simulink model "basic_cosimulation_c_1_sm_master"  (R2021b)
settings: Solver=ode4  StartTime=0.0  StopTime=inf  FixedStep=5e-05  RelTol=1e-3  EnableMultiTasking=on
PostLoadFcn:
  | %
  | % Script for validation of swtiching model design with it's respective
  | % average model.
  | %
  | % Here it is presented the design of the inverter to the 6 kW Fuel Cell
  | % model.
  | 
  | %%% Initialization %%%
  | 
  | 
  | % ------------------------------------- %
  | % ---------- Inverter Design ---------- %
  | % ------------------------------------- %
  | 
  | %%%% Nominal Parameters %%%%
  | 
  | Pnom = 50e3;                                        % Nominal Power
  | Vdc = 400;                                          % DC Voltage - Boost
  | m = 0.6;                                            % Modulation Index
  | Vnom_peak = m*Vdc/2;                                % Peak Voltage
  | Vnom_rms = Vnom_peak/sqrt(2);                       % Rms Voltage
  | FP_min = 0.9;                                       % For Reactive Power
  |                                                     % Compensation
  | Snom = Pnom/FP_min;                                 % Apparent Power
  | Irms = Pnom/(sqrt(3)*Vnom_rms);                     % Rms Curren
  | Inom_peak = Irms*sqrt(2);                           % Peak Current
  | Zbase = Vnom_peak/Inom_peak;                        % Base Impedance
  | f = 60;                                             % Nominal Frequency
  | wnom = 2*pi*60;                                     % Angular Frequency
  | 
  | % ------------------------- %
  | % Inverter LC Filter Design %
  | % ------------------------- %
  | 
  | fsw_inv = 96*60;                                    % Switching Frequency must be a multiple of the nominal frequency
  |                                                      % for proper operation of the Artemis Block
  | ripple_inv = 0.03;
  | L_inv = ((Vdc/2)-Vnom_peak)*(1/fsw_inv)/(ripple_inv*Inom_peak);
  | 
  | % - Capacitor
  | fres = 420;                                         % Filters Ressonant Frequency
  | 
  | Cf = 1/(4*L_inv*(pi^2)*(fres^2));                % Filter Capacitor
  | Rf = 1/(wnom*Cf*50);                                % Damping Resistor
  | 
  | % --- Sample Time --- %
  | 
  | Tsw = 0.00050;
  | Ts = Tsw/10;
  | 
  | % ---------------------- %
  | % Current Control Design %
  | % ---------------------- %
  | 
  | Ron = 0.001;                                        % IGBT Resistance
  | tau_i = 1e-3;                                       % Responde Time
  | kp_current = L_inv/tau_i;                           % PI Proportional Gain
  | ki_current = (Ron)/tau_i;                           % PI Integral Gain
  | 
  | decouple = (wnom*L_inv);                            % Decoupling Gain
InitFcn:
  | %
  | % Script for validation of swtiching model design with it's respective
  | % average model.
  | %
  | % Here it is presented the design of the inverter to the 6 kW Fuel Cell
  | % model.
  | 
  | %%% Initialization %%%
  | 
  | 
  | % ------------------------------------- %
  | % ---------- Inverter Design ---------- %
  | % ------------------------------------- %
  | 
  | %%%% Nominal Parameters %%%%
  | 
  | Pnom = 50e3;                                        % Nominal Power
  | Vdc = 400;                                          % DC Voltage - Boost
  | m = 0.6;                                            % Modulation Index
  | Vnom_peak = m*Vdc/2;                                % Peak Voltage
  | Vnom_rms = Vnom_peak/sqrt(2);                       % Rms Voltage
  | FP_min = 0.9;                                       % For Reactive Power
  |                                                     % Compensation
  | Snom = Pnom/FP_min;                                 % Apparent Power
  | Irms = Pnom/(sqrt(3)*Vnom_rms);                     % Rms Curren
  | Inom_peak = Irms*sqrt(2);                           % Peak Current
  | Zbase = Vnom_peak/Inom_peak;                        % Base Impedance
  | f = 60;                                             % Nominal Frequency
  | wnom = 2*pi*60;                                     % Angular Frequency
  | 
  | % ------------------------- %
  | % Inverter LC Filter Design %
  | % ------------------------- %
  | 
  | fsw_inv = 96*60;                                    % Switching Frequency must be a multiple of the nominal frequency
  |                                                      % for proper operation of the Artemis Block
  | ripple_inv = 0.03;
  | L_inv = ((Vdc/2)-Vnom_peak)*(1/fsw_inv)/(ripple_inv*Inom_peak);
  | 
  | % - Capacitor
  | fres = 420;                                         % Filters Ressonant Frequency
  | 
  | Cf = 1/(4*L_inv*(pi^2)*(fres^2));                % Filter Capacitor
  | Rf = 1/(wnom*Cf*50);                                % Damping Resistor
  | 
  | % --- Sample Time --- %
  | 
  | Tsw = 0.00050;
  | Ts = Tsw/10;
  | 
  | % ---------------------- %
  | % Current Control Design %
  | % ---------------------- %
  | 
  | Ron = 0.001;                                        % IGBT Resistance
  | tau_i = 1e-3;                                       % Responde Time
  | kp_current = L_inv/tau_i;                           % PI Proportional Gain
  | ki_current = (Ron)/tau_i;                           % PI Integral Gain
  | 
  | decouple = (wnom*L_inv);                            % Decoupling Gain
undefined symbols (not defined in the file or in its folder): D1, Delta, DiscIntNeverNeededParam, IP, j, ph, sps, UDP
libraries: spsCurrentMeasurementLib x25, spsControlledVoltageSourceLib x21, rtlab x16, spsGroundLib x13, spsThreePhaseSeriesRLCBranchLib x13, spsControlledCurrentSourceLib x11, spsVoltageMeasurementLib x10, simulink x8, rteventslib x8, powerlib_meascontrol x7, spsThreePhaseVIMeasurementLib x4, ssn_inverter_model x4
(part 1 of 5)
Description:
  | Circuits used for co-simulation studies.
settings Model: ARTEMISmethode_block_infos=$$__separator__$$basic_cosimulation_c_1_sm_master/ARTEMIS Guide$$__separator__$$  Creator=Antero  LastModifiedBy=Antero
settings SolverCC: AlgebraicLoopSolver=TrustRegion
settings DataIOCC: LimitDataPoints=on  SaveFormat=Array  SignalLoggingSaveFormat=ModelDataLogs  SaveOutput=off  SaveTime=off  ReturnWorkspaceOutputs=off  SignalLoggingName=sigsOut
settings OptimizationCC: BlockReduction=off  BooleanDataType=off  OptimizeBlockIOStorage=off  BufferReuse=off  ExpressionFolding=off  LocalBlockOutputs=off  InitFltsAndDblsToZero=on  LifeSpan=inf
settings DebuggingCC: SaveWithParameterizedLinksMsg=none  UnderspecifiedInitializationDetection=Classic  MergeDetectMultiDrivingBlocksExec=none  SignalResolutionControl=TryResolveAllWithWarning  MultiTaskDSMMsg=warning  MultiTaskCondExecSysMsg=none  FcnCallInpInsideContextMsg=warning  SFUnexpectedBacktrackingDiag=warning  SFNoUnconditionalDefaultTransitionDiag=warning  SFExecutionAtInitializationDiag=none  SFMachineParentedDataDiag=warning  ArithmeticOperatorsInVariantConditions=warning
settings HardwareCC: ProdBitPerPointer=32  ProdBitPerSizeT=32  ProdBitPerPtrDiffT=32  ProdLargestAtomicFloat=None  ProdIntDivRoundTo=Undefined  ProdEndianess=Unspecified  ProdWordSize=32  ProdHWDeviceType=32-bit Generic  TargetBitPerPointer=64  TargetBitPerSizeT=64  TargetBitPerPtrDiffT=64  TargetLongLongMode=on  TargetIntDivRoundTo=Zero  TargetEndianess=LittleEndian  TargetWordSize=64  TargetHWDeviceType=MATLAB Host  ProdEqTarget=off
settings ModelReferenceCC: PropagateSignalLabelsOutOfModel=off
settings SFSimCC: SimUseLocalCustomCode=off  CustomCodeUndefinedFunction=UseInterfaceOnly
settings RTWCC: GenCodeOnly=on  RTWUseLocalCustomCode=off
settings CodeAppCC: StateflowObjectComments=on
settings GRTTargetCC: TargetFcnLib=ansi_tfl_tmw.mat  TargetLangStandard=C89/C90 (ANSI)  CombineOutputUpdateFcns=off  GRTInterface=on
settings ConfigComp: CovMetricSettings=dw  CovSaveCumulativeToWorkspaceVar=on  CovSaveSingleToWorkspaceVar=on  CovExternalEMLEnable=off

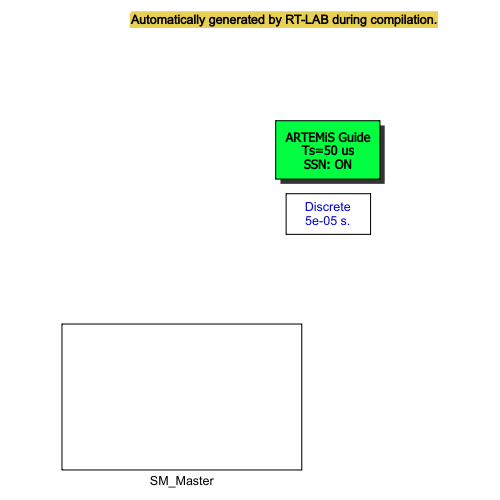
[thumbnail: Simulink's stored preview of the top-level diagram]
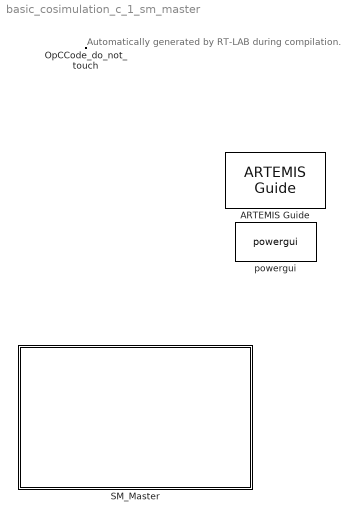
== system basic_cosimulation_c_1_sm_master ==
  note: Automatically generated by RT-LAB during compilation.
  ARTEMIS Guide : artemis/ARTEMIS/ARTEMIS Guide  Tag=art7.5  Description=New ARTEMiS block v 7.5b (R2015b+)  lock=on  Ts=Ts  ssn=on  opt=art5  dyna=off  nb_perm=4  RT_fullcomp=off  ssn_itvc=off  ssn_ivic=off  ssn_ext=off  ssn_solver=Art5  iter_type=iSWITCH and iMOV only (default)  ssn_ImpulseLoopBlockedStateUpdate=5  ssn_mov_iter_number=5  ssn_switch_iter_number=3  ssn_lu_or_ldlt=LU (more robust)  ssn_nib_type_verify=on  ssn_use_lu=on  ssn_use_ldlt=off  ssn_impulse=on  ssn_quasimpulse=off  ssn_impulse_loop=5  paraExtinctionThy=off  Thy_Impulse=on  dtc=Off  dtc_opt=normal  ao=off  simtype=off  ct_mac=off  lin_mov=off  lsp=[0.001 2]  spike_skip=Disabled  dtc_extra=1  dtc_sws=normal  dtc_pied=0.5  SPSRulesBlock=SPSRules  tre=off  ctmm=off  LF=off  dpl_type=ARTEMiS DPL  rlc_type=off  custom_type=off  para=on  ssn_full_iteration=off  ssn_init_cond=block only
  OpCCode_do_not_touch : opal_lib/Communication/OpCCode  SystemSampleTime=-1  VariantActivationTime=update diagram  Latency=0  AutoFrameSizeCalculation=off
  SM_Master : Subsystem
  powergui : spspowerguiLib/powergui  SimulationMode=Discrete  SampleTime=5e-05  frequency=60  Iterations=50  frequencyindice=0  Pbase=100e6  ErrMax=1e-4  UnitsV=kV  UnitsW=MW  buscounter=0  FunctionMessages=off  echomessages=off  EnableUseOfTLC=off  CurrentSourceSwitches=off  DisableSnubberDevices=off  DisableRonSwitches=off  DisableVfSwitches=off  DisplayEquations=off  AutomaticDiscreteSolvers=off  SolverType=Tustin/Backward Euler (TBE)  Interpol=off  ExternalGateDelay=off  methode=off  Ts=100  x0status=blocks  SPID=on  SwTol=0  HookPort=off  NonlinearTolerance=1e-4  nMaxIteration=100  ContinueOnMaxIteration=off  RestoreLinks=warning  ResistiveCurrentMeasurement=off  Frange=[0:2:500]  Ylog=off  Xlog=on  ShowGrid=off  save=off  variable=ZData  structure=0  ZoomFFT=off  StartTime=0.0  cycles=1  DisplayStyle=1  fundamental=60  FreqAxis=off  MaxFrequency=1000  frequencyindicesteady=1  RmsSteady=1  display=off

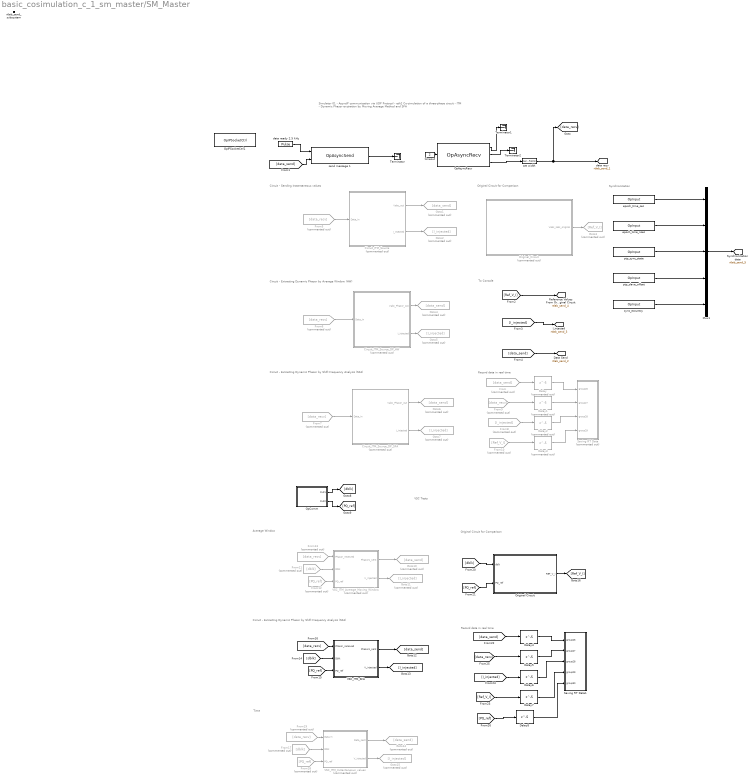
== system basic_cosimulation_c_1_sm_master/SM_Master ==
  note: Synchronization
  note: VSC Tests
  note: Circuit - Sending Instantaneous values
  note: To Console
  note: Circuit - Extracting Dynamic Phasor by Shift Frequency Analysis (SFA)
  note: Circuit - Extracting Dynamic Phasor by Average Window (AW)
  note: Original Circuit for Comparison
  note: Record data in real time
  note: Simulator 01 - AsyncIP communication via UDP Protocol - eth2
      |
      | Co-simulation of a three-phase circuit - ITM - Dynamic Phasor exctration by Moving Average Method and SFA
  note: Average Window
  note: Original Circuit for Comparison
  note: Circuit - Extracting Dynamic Phasor by Shift Frequency Analysis (SFA)
  note: Time
  note: Record data in real time
  Circuit_ITM_Source : Subsystem  Commented=on
  Circuit_ITM_Source_DP_AW : Subsystem  Commented=on
  Circuit_ITM_Source_DP_SFA : Subsystem  Commented=on
  Delay{,1..3} (4 alike) : Delay  Commented=on  DelayLength=5  InitialCondition=0  UseCircularBuffer=on
  Delay{4..8} (5 alike) : Delay  DelayLength=5  InitialCondition=0  UseCircularBuffer=on
  From : From  Commented=on  GotoTag=data_send
  From10 : From  Commented=on  GotoTag=Ref_V_I
  From11 : From  Commented=on  GotoTag=dblk
  From12 : From  Commented=on  GotoTag=PQ_ref
  From{5..7,9,13,19} (6 alike) : From  Commented=on  GotoTag=data_recv
  From17 : From  Commented=on  GotoTag=dblk
  From18 : From  Commented=on  GotoTag=PQ_ref
  From8 : From  Commented=on  GotoTag=I_injected
  Goto{1,4,6,10,14} (5 alike) : Goto  Commented=on  GotoTag=data_send
  Goto{2,5,7,11,15} (5 alike) : Goto  Commented=on  GotoTag=I_injected
  Goto3 : Goto  Commented=on  GotoTag=Ref_V_I
  Mux1 : Mux  Inputs=5
  OpAsyncRecv : rtlab/Communication/Asynchronous/OpAsyncRecv  ctl_id=1  recv_id=1  enable_param=off  fp1=1  fp2=2  fp3=3  fp4=4  fp5=5  sp1=string1  sp2=string2  sp3=string3  sp4=string4  sp5=string5  fp6=6  fp7=7
      settings: SourceProductName=RT-LAB
  OpComm : Subsystem
      mask init:
      | opmaskdisplay('maskdisplay_block',gcb,'disp(''OpComm'')');
      mask Display:
      | patch([0 0.5 0.7 0],[1 1 0 0],[0.7 0.75 0.9]);
      | patch([1 0.53 0.73 1],[1 1 0 0],[1 0.8 0.7]);
      | plot([0 0 1 1 0],[0 1 1 0 0]);
      | disp('OpComm')
  OpIPSocketCtrl1 : rtio_generic_ip/OpIPSocketCtrl  ctl_id=1  proto=UDP/IP  ip_addr_remote=192.168.10.16  ip_port_remote=23002  ip_port_local=23001  ip_addr_mcast=0.0.0.0  exe_name=AsyncIP
      settings: SourceProductName=RT-LAB I/O
  Original Circuit : Subsystem
  Original_Circuit : Subsystem  Commented=on
  Saving RT Data : Subsystem  Commented=on  mask{Ts=Ts, varname26=data_send, Filename26=data_send.mat, nls26=3, ld26=10, varname27=data_recv, Filename27=data_recv.mat, nls27=3, ld27=10, varname28=I_injected, Filename28=I_injected.mat, nls28=3, ld28=10, varname29=Ref_V_I, Filename29=Ref_V_I.mat, nls29=6, ld29=10, varname30=, Filename30=, nls30=0, ld30=0}
      mask prompts: Ts "Ts (s)"; varname26 "Variable name"; Filename26 "FileName"; nls26 "Number of logged signals"; ld26 "Logging duration (s)"; varname27 "Variable name"; Filename27 "FileName"; nls27 "Number of logged signals"; ld27 "Logging duration (s)"; varname28 "Variable name"; Filename28 "FileName"; nls28 "Number of logged signals"; ld28 "Logging duration (s)"; varname29 "Variable name"; Filename29 "FileName"; nls29 "Number of logged signals"; ld29 "Logging duration (s)"; varname30 "Variable name"; Filename30 "FileName"; nls30 "Number of logged signals"; ld30 "Logging duration (s)"
      mask help: This block contains the 5 groups of OpWriteFile (26, 27, 28 29 and 30) blocks that write signals to a binary file (.mat), files that are in the binary data container format that MATLAB uses.
      mask TypeOptions varname26: OpWriteFile26/varname
      mask TypeOptions Filename26: OpWriteFile26/Filename
      mask TypeOptions varname27: OpWriteFile27/varname
      mask TypeOptions Filename27: OpWriteFile27/Filename
      mask TypeOptions varname28: OpWriteFile28/varname
      mask TypeOptions Filename28: OpWriteFile28/Filename
      mask TypeOptions varname29: OpWriteFile29/varname
      mask TypeOptions Filename29: OpWriteFile29/Filename
      mask TypeOptions varname30: OpWriteFile30/varname
      mask TypeOptions Filename30: OpWriteFile30/Filename
      mask DialogControl DescGroupVar Prompt: Saving RT Data
      mask DialogControl Container4 Prompt: Group 26
      mask DialogControl Container9 Prompt: Group 27
      mask DialogControl Container10 Prompt: Group 28
      mask DialogControl Container11 Prompt: Group 29
      mask DialogControl Container12 Prompt: Group 30
  Saving RT Data1 : Subsystem  mask{Ts=Ts, varname26=data_send, Filename26=data_send.mat, nls26=6, ld26=20, varname27=data_recv, Filename27=data_recv.mat, nls27=6, ld27=20, varname28=V_injected, Filename28=V_injected.mat, nls28=3, ld28=20, varname29=Ref_V_I, Filename29=Ref_V_I.mat, nls29=6, ld29=20, varname30=PQ_ref, Filename30=PQ_ref.mat, nls30=2, ld30=20}
      mask prompts: Ts "Ts (s)"; varname26 "Variable name"; Filename26 "FileName"; nls26 "Number of logged signals"; ld26 "Logging duration (s)"; varname27 "Variable name"; Filename27 "FileName"; nls27 "Number of logged signals"; ld27 "Logging duration (s)"; varname28 "Variable name"; Filename28 "FileName"; nls28 "Number of logged signals"; ld28 "Logging duration (s)"; varname29 "Variable name"; Filename29 "FileName"; nls29 "Number of logged signals"; ld29 "Logging duration (s)"; varname30 "Variable name"; Filename30 "FileName"; nls30 "Number of logged signals"; ld30 "Logging duration (s)"
      mask help: This block contains the 5 groups of OpWriteFile (26, 27, 28 29 and 30) blocks that write signals to a binary file (.mat), files that are in the binary data container format that MATLAB uses.
      mask TypeOptions varname26: OpWriteFile26/varname
      mask TypeOptions Filename26: OpWriteFile26/Filename
      mask TypeOptions varname27: OpWriteFile27/varname
      mask TypeOptions Filename27: OpWriteFile27/Filename
      mask TypeOptions varname28: OpWriteFile28/varname
      mask TypeOptions Filename28: OpWriteFile28/Filename
      mask TypeOptions varname29: OpWriteFile29/varname
      mask TypeOptions Filename29: OpWriteFile29/Filename
      mask TypeOptions varname30: OpWriteFile30/varname
      mask TypeOptions Filename30: OpWriteFile30/Filename
      mask DialogControl DescGroupVar Prompt: Saving RT Data
      mask DialogControl Container4 Prompt: Group 26
      mask DialogControl Container9 Prompt: Group 27
      mask DialogControl Container10 Prompt: Group 28
      mask DialogControl Container11 Prompt: Group 29
      mask DialogControl Container12 Prompt: Group 30
  Terminator : Terminator
  Terminator1 : Terminator
  Terminator2 : Terminator
  VSC_ITM_Average_Moving_Window : Subsystem  Commented=on
  VSC_ITM_Instantaneous_values : Subsystem  Commented=on
  VSC_ITM_SFA : Subsystem
  data ready 2.5 kHz : DiscretePulseGenerator  PulseWidth=2  SampleTime=Ts
  epoch_time_nsec : rtlab/OpInput  identifier_use=[]  identifier_hide=epoch_time_nsec  nb_parents_identifier=0  passthrough=off  init_value=0  value_type=double  create_alias=on
      settings: SourceProductName=RT-LAB
  epoch_time_sec : rtlab/OpInput  identifier_use=[]  identifier_hide=epoch_time_sec  nb_parents_identifier=0  passthrough=off  init_value=0  value_type=double  create_alias=on
      settings: SourceProductName=RT-LAB
  ptp_slave_offset : rtlab/OpInput  identifier_use=[]  identifier_hide=ptp_slave_offset  nb_parents_identifier=0  passthrough=off  init_value=0  value_type=double  create_alias=on
      settings: SourceProductName=RT-LAB
  ptp_sync_state : rtlab/OpInput  identifier_use=[]  identifier_hide=ptp_sync_state  nb_parents_identifier=0  passthrough=off  init_value=0  value_type=double  create_alias=on
      settings: SourceProductName=RT-LAB
  rtlab_send_subsystem : Subsystem  Priority=-100
      mask Display: text(0,0,'');
  send message 1 : rtlab/Communication/Asynchronous/OpAsyncSend  ctl_id=1  send_id=1  mode=DONT_NEED_REPLY  enable_param=off  fp1=1  fp2=2  fp3=3  fp4=4  fp5=5  sp1=string1  sp2=string2  sp3=string3  sp4=string4  sp5=string5
      settings: SourceProductName=RT-LAB
  set width : SignalSpecification  Dimensions=6  SampleTime=Ts
  sync_accuracy : rtlab/OpInput  identifier_use=[]  identifier_hide=sync_accuracy  nb_parents_identifier=0  passthrough=off  init_value=0  value_type=double  create_alias=on
      settings: SourceProductName=RT-LAB
  timeout : Constant  Value=2
  tag scope: rtlab_send_1=global, rtlab_send_2=global, rtlab_send_3=global, rtlab_send_4=global, rtlab_send_5=global
  wires:
  set width/1 -> [rtlab_send_1], [data_recv]
  send message 1/1 -> Terminator/1
  OpAsyncRecv/2 -> Terminator2/1
  timeout/1 -> OpAsyncRecv/1
  data ready 2.5 kHz/1 -> send message 1/1
  OpAsyncRecv/3 -> set width/1
  OpAsyncRecv/1 -> Terminator1/1
  [I_injected] -> [rtlab_send_3]
  From6/1 -> Circuit_ITM_Source_DP_AW/1(Data_In)
  [Ref_V_I] -> [rtlab_send_4]
  [data_send] -> [rtlab_send_2]
  Circuit_ITM_Source_DP_SFA/1(Vabc_Phasor_out) -> Goto6/1
  Circuit_ITM_Source_DP_AW/1(Vabc_Phasor_out) -> Goto4/1
  Circuit_ITM_Source/1(Vabc_out) -> Goto1/1
  Original_Circuit/1(Vabc_Iabc_original) -> Goto3/1
  From5/1 -> Circuit_ITM_Source/1(Data_In)
  Circuit_ITM_Source/2(I_injected) -> Goto2/1
  From7/1 -> Circuit_ITM_Source_DP_SFA/1(Data_In)
  Circuit_ITM_Source_DP_SFA/2(I_injected) -> Goto7/1
  Circuit_ITM_Source_DP_AW/2(I_injected) -> Goto5/1
  From8/1 -> Delay2/1
  From10/1 -> Delay3/1
  From9/1 -> Delay1/1
  From/1 -> Delay/1
  Delay/1 -> Saving RT Data/1(group26)
  Delay1/1 -> Saving RT Data/2(group27)
  Delay2/1 -> Saving RT Data/3(group28)
  Delay3/1 -> Saving RT Data/4(group29)
  OpComm/1(Out1) -> [dblk]
  OpComm/2(Out2) -> [PQ_ref]
  From11/1 -> VSC_ITM_Average_Moving_Window/2(Dblk)
  From12/1 -> VSC_ITM_Average_Moving_Window/3(PQ_ref)
  From13/1 -> VSC_ITM_Average_Moving_Window/1(Phasor_received)
  VSC_ITM_Average_Moving_Window/1(Phasors_sent) -> Goto10/1
  VSC_ITM_Average_Moving_Window/2(V_injected) -> Goto11/1
  VSC_ITM_SFA/1(Phasors_sent) -> [data_send]
  [PQ_ref] -> VSC_ITM_SFA/3(PQ_ref)
  [dblk] -> VSC_ITM_SFA/2(Dblk)
  [data_recv] -> VSC_ITM_SFA/1(Phasor_received)
  VSC_ITM_SFA/2(V_injected) -> [I_injected]
  VSC_ITM_Instantaneous_values/1(Data_sent) -> Goto14/1
  From18/1 -> VSC_ITM_Instantaneous_values/3(PQ_ref)
  From17/1 -> VSC_ITM_Instantaneous_values/2(Dblk)
  From19/1 -> VSC_ITM_Instantaneous_values/1(Data in)
  VSC_ITM_Instantaneous_values/2(V_injected) -> Goto15/1
  [dblk] -> Original Circuit/1(dblk)
  [data_recv] -> Delay5/1
  Delay6/1 -> Saving RT Data1/3(group28)
  [Ref_V_I] -> Delay7/1
  Delay5/1 -> Saving RT Data1/2(group27)
  [I_injected] -> Delay6/1
  Delay4/1 -> Saving RT Data1/1(group26)
  [data_send] -> Delay4/1
  Delay7/1 -> Saving RT Data1/4(group29)
  [PQ_ref] -> Original Circuit/2(PQ_ref)
  [PQ_ref] -> Delay8/1
  Delay8/1 -> Saving RT Data1/5(group30)
  Original Circuit/1(REF_V_I) -> [Ref_V_I]
  ptp_slave_offset/1 -> Mux1/4
  Mux1/1 -> [rtlab_send_5]
  ptp_sync_state/1 -> Mux1/3
  sync_accuracy/1 -> Mux1/5
  epoch_time_sec/1 -> Mux1/1
  epoch_time_nsec/1 -> Mux1/2
  [data_send] -> send message 1/2

== system basic_cosimulation_c_1_sm_master/SM_Master/Circuit_ITM_Source ==
  Data_In : Inport
  Amplitude : Step  Time=3  Before=220*sqrt(2/3)  After=220*sqrt(2/3)  SampleTime=Ts
  "Amplitude1 " : Step  Time=4  After=0  SampleTime=Ts
  Controllable Voltage Source 1 : Subsystem
  Demux : Demux  Outputs=3
  Freq : Step  Time=2.8  After=0  SampleTime=Ts
  Freq Ref : Step  Time=2  Before=60  After=60  SampleTime=Ts
  Phase Ref : Constant  Value=0  SampleTime=Ts
  Sum : Sum  Inputs=-+|
  Sum1 : Sum  Inputs=|+-
  Three-Phase Series RLC Branch1 : spsThreePhaseSeriesRLCBranchLib/Three-Phase Series RLC Branch  LConnTagsString=A|B|C  RConnTagsString=A|B|C  BranchType=R  Resistance=2  Inductance=1e-3  Capacitance=1e-6  Measurements=None
  Three-Phase V-I Measurement : spsThreePhaseVIMeasurementLib/Three-Phase V-I Measurement  VoltageMeasurement=phase-to-ground  SetLabelV=off  LabelV=Vabc  Vpu=off  VpuLL=off  CurrentMeasurement=yes  SetLabelI=off  LabelI=Iabc  Ipu=off  Pbase=100e6  Vbase=25e3  OutputType=Complex  PhasorSimulation=off  PSBequivalent=0
  Three-Phase Controlled Y-Connected Current Source : Subsystem
      settings: PortSchema="{\"entries\":[{\"content\":{\"sides\":[{\"content\":{\"connectorIds\":[\"LConn1\",\"LConn2\",\"LConn3\"]},\"type\":\"ConnectorPlacement.EquallySpacedRectSide\",\"uuid\":\"a8a67328-a09d-4495-b33c-aaf3ca0795cb\"},{\"content\":{\"connectorIds\":[\"In1\",\"In2\",\"In3\"],\"side\":\"RIGHT\"},\"type\":\"ConnectorPlacement.EquallySpacedRectSide\",\"uuid\":\"ca8d97e2-0dea-49aa-8cb7-235b4eace1f8\"},{\"content\":{\"connectorIds\":[],\"side\":\"TOP\"},\"type\":\"ConnectorPlacement.EquallySpacedRectSide\",\"uuid\":\"ab6aade9-1d27-4135-8ce1-c4358d4ecc87\"}]},\"type\":\"ConnectorPlacement.EquallySpacedConnector\",\"uuid\":\"205b5c38-55ea-4d68-a706-de660c21807c\"}],\"packageUris\":[\"http://schema.mathworks.com/mf0/Connector/19700101\"],\"version\":\"1.0\"}"
  Vabc_out : Outport
  I_injected : Outport  Port=2
  wires:
  Demux/1 -> Three-Phase Controlled Y-Connected Current Source/1(Ia)
  Demux/2 -> Three-Phase Controlled Y-Connected Current Source/2(Ib)
  Demux/3 -> Three-Phase Controlled Y-Connected Current Source/3(Ic)
  Data_In/1 -> Demux/1, I_injected/1
  Three-Phase V-I Measurement/1 -> Vabc_out/1
  "Amplitude1 "/1 -> Sum/1
  Freq Ref/1 -> Sum1/1
  Sum1/1 -> Controllable Voltage Source 1/3(Frequency [Hz])
  Freq/1 -> Sum1/2
  Amplitude/1 -> Sum/2
  Phase Ref/1 -> Controllable Voltage Source 1/2(Phase [Deg])
  Sum/1 -> Controllable Voltage Source 1/1(Amplitude [V])
  connections:
  Three-Phase Series RLC Branch1/RConn2 -- Three-Phase V-I Measurement/LConn2
  Three-Phase V-I Measurement/LConn3 -- Three-Phase Series RLC Branch1/RConn3
  Three-Phase V-I Measurement/LConn1 -- Three-Phase Series RLC Branch1/RConn1
  Three-Phase Controlled Y-Connected Current Source/LConn1 -- Three-Phase V-I Measurement/RConn1
  Three-Phase V-I Measurement/RConn2 -- Three-Phase Controlled Y-Connected Current Source/LConn2
  Three-Phase V-I Measurement/RConn3 -- Three-Phase Controlled Y-Connected Current Source/LConn3
  Controllable Voltage Source 1/RConn2 -- Three-Phase Series RLC Branch1/LConn2
  Controllable Voltage Source 1/RConn1 -- Three-Phase Series RLC Branch1/LConn1
  Controllable Voltage Source 1/RConn3 -- Three-Phase Series RLC Branch1/LConn3

== system basic_cosimulation_c_1_sm_master/SM_Master/Circuit_ITM_Source_DP_AW ==
  Data_In : Inport
  AC Voltage Source : spsACVoltageSourceLib/AC Voltage Source  Commented=on  Amplitude=100  Phase=0  Frequency=60  SampleTime=0  Measurements=None  BusType=swing  Pref=10e3  Qref=0  Qmin=-inf  Qmax=+inf
  Amplitude : Step  Time=3  Before=220*sqrt(2/3)  After=220*sqrt(2/3)*0.8  SampleTime=Ts
  "Amplitude1 " : Step  Time=4  After=-220*sqrt(2/3)*0.2  SampleTime=Ts
  Constant : Constant  Commented=on  Value=5/60  SampleTime=Ts
  "Controllable Voltage Source " : Subsystem
  Controlled Current Source : spsControlledCurrentSourceLib/Controlled Current Source  Commented=on  Initialize=on  Source_Type=AC  Amplitude=0  Phase=0  Frequency=0  Measurements=None
  DP - > EMT : Subsystem
  DP --> EMT : Subsystem  Commented=on
  Demux1 : Demux  Outputs=3
  Digital Clock : DigitalClock  Commented=on  SampleTime=Ts
  Dynamic Phasor coeficientes extraction : Subsystem
  Dynamic Phasor coeficients extraction : Subsystem  Commented=on
  Freq : Step  Time=2.8  After=-2  SampleTime=Ts
  Freq Ref : Step  Time=2  Before=60  After=58  SampleTime=Ts
  GreaterThan : RelationalOperator  Commented=on  Operator=>  OutDataTypeStr=boolean  RndMeth=Simplest
  Ground1 : spsGroundLib/Ground  Commented=on  LConnTagsString=a
  Mux : Mux  Inputs=3
  Mux1 : Mux  Inputs=3
  Phase Ref : Constant  Value=0  SampleTime=Ts
  Series RLC Branch : spsSeriesRLCBranchLib/Series RLC Branch  Commented=on  LConnTagsString=__new0  RConnTagsString=__new0  BranchType=R  Resistance=0.5  Inductance=1e-3  SetiL0=off  InitialCurrent=0  Capacitance=1e-6  Setx0=off  InitialVoltage=0  Measurements=None
  Subsystem : Subsystem  Commented=on
  Sum : Sum  Inputs=-+|
  Sum1 : Sum  Inputs=|+-
  Three-Phase Series RLC Branch1 : spsThreePhaseSeriesRLCBranchLib/Three-Phase Series RLC Branch  LConnTagsString=A|B|C  RConnTagsString=A|B|C  BranchType=R  Resistance=2  Inductance=1e-3  Capacitance=1e-6  Measurements=None
  Three-Phase V-I Measurement : spsThreePhaseVIMeasurementLib/Three-Phase V-I Measurement  VoltageMeasurement=phase-to-ground  SetLabelV=off  LabelV=Vabc  Vpu=off  VpuLL=off  CurrentMeasurement=yes  SetLabelI=off  LabelI=Iabc  Ipu=off  Pbase=100e6  Vbase=25e3  OutputType=Complex  PhasorSimulation=off  PSBequivalent=0
  Three-Phase Controlled Y-Connected Current Source : Subsystem
      settings: PortSchema="{\"entries\":[{\"content\":{\"sides\":[{\"content\":{\"connectorIds\":[\"LConn1\",\"LConn2\",\"LConn3\"]},\"type\":\"ConnectorPlacement.EquallySpacedRectSide\",\"uuid\":\"a8a67328-a09d-4495-b33c-aaf3ca0795cb\"},{\"content\":{\"connectorIds\":[\"In1\",\"In2\",\"In3\"],\"side\":\"RIGHT\"},\"type\":\"ConnectorPlacement.EquallySpacedRectSide\",\"uuid\":\"ca8d97e2-0dea-49aa-8cb7-235b4eace1f8\"},{\"content\":{\"connectorIds\":[],\"side\":\"TOP\"},\"type\":\"ConnectorPlacement.EquallySpacedRectSide\",\"uuid\":\"ab6aade9-1d27-4135-8ce1-c4358d4ecc87\"}]},\"type\":\"ConnectorPlacement.EquallySpacedConnector\",\"uuid\":\"205b5c38-55ea-4d68-a706-de660c21807c\"}],\"packageUris\":[\"http://schema.mathworks.com/mf0/Connector/19700101\"],\"version\":\"1.0\"}"
  Voltage Measurement : spsVoltageMeasurementLib/Voltage Measurement  Commented=on  PhasorSimulation=off  OutputType=Complex  PSBequivalent=0
  Vabc_Phasor_out : Outport
  I_injected : Outport  Port=2
  wires:
  DP --> EMT/1(I_injected) -> Controlled Current Source/1
  Voltage Measurement/1 -> Dynamic Phasor coeficients extraction/1(EMT Signal)
  Dynamic Phasor coeficients extraction/1(Mag) -> ?
  Dynamic Phasor coeficients extraction/2(Phase) -> ?
  Data_In/1 -> Demux1/1
  Three-Phase V-I Measurement/1 -> Dynamic Phasor coeficientes extraction/1(EMT_Signal)
  Dynamic Phasor coeficientes extraction/3(Phasor_C) -> Mux/3
  Dynamic Phasor coeficientes extraction/2(Phasor_B) -> Mux/2
  Dynamic Phasor coeficientes extraction/1(Phasor_A) -> Mux/1
  Mux/1 -> Vabc_Phasor_out/1
  Demux1/1 -> DP - > EMT/1(Phasor_A)
  Demux1/2 -> DP - > EMT/2(Phasor_B)
  Demux1/3 -> DP - > EMT/3(Phasor_C)
  DP - > EMT/2(Sinal_B) -> Mux1/2, Three-Phase Controlled Y-Connected Current Source/2(Ib)
  DP - > EMT/1(Sinal_A) -> Mux1/1, Three-Phase Controlled Y-Connected Current Source/1(Ia)
  DP - > EMT/3(Sinal_C) -> Mux1/3, Three-Phase Controlled Y-Connected Current Source/3(Ic)
  Mux1/1 -> I_injected/1
  Digital Clock/1 -> GreaterThan/1
  Constant/1 -> GreaterThan/2
  GreaterThan/1 -> ?
  Freq/1 -> Sum1/2
  Amplitude/1 -> Sum/2
  Sum/1 -> "Controllable Voltage Source "/1(Amplitude [V])
  Freq Ref/1 -> Sum1/1
  "Amplitude1 "/1 -> Sum/1
  Sum1/1 -> "Controllable Voltage Source "/3(Frequency [Hz])
  Phase Ref/1 -> "Controllable Voltage Source "/2(Phase [Deg])
  connections:
  AC Voltage Source/RConn1 -- Series RLC Branch/LConn1
  AC Voltage Source/LConn1 -- Controlled Current Source/RConn1 -- Voltage Measurement/LConn2 -- Ground1/LConn1
  Series RLC Branch/RConn1 -- Voltage Measurement/LConn1 -- Controlled Current Source/LConn1
  Three-Phase Series RLC Branch1/RConn2 -- Three-Phase V-I Measurement/LConn2
  Three-Phase V-I Measurement/LConn3 -- Three-Phase Series RLC Branch1/RConn3
  Three-Phase V-I Measurement/LConn1 -- Three-Phase Series RLC Branch1/RConn1
  Three-Phase Controlled Y-Connected Current Source/LConn1 -- Three-Phase V-I Measurement/RConn1
  Three-Phase V-I Measurement/RConn2 -- Three-Phase Controlled Y-Connected Current Source/LConn2
  Three-Phase V-I Measurement/RConn3 -- Three-Phase Controlled Y-Connected Current Source/LConn3
  "Controllable Voltage Source "/RConn1 -- Three-Phase Series RLC Branch1/LConn1
  Three-Phase Series RLC Branch1/LConn2 -- "Controllable Voltage Source "/RConn2
  Three-Phase Series RLC Branch1/LConn3 -- "Controllable Voltage Source "/RConn3

== system basic_cosimulation_c_1_sm_master/SM_Master/Circuit_ITM_Source_DP_SFA ==
  Data_In : Inport
  AC Voltage Source : spsACVoltageSourceLib/AC Voltage Source  Commented=on  Amplitude=100  Phase=0  Frequency=60  SampleTime=0  Measurements=None  BusType=swing  Pref=10e3  Qref=0  Qmin=-inf  Qmax=+inf
  Amplitude : Step  Time=3  Before=220*sqrt(2/3)  After=220*sqrt(2/3)*0.8  SampleTime=Ts
  "Amplitude1 " : Step  Time=4  After=-220*sqrt(2/3)*0.2  SampleTime=Ts
  "Controllable Voltage Source " : Subsystem
  Controlled Current Source : spsControlledCurrentSourceLib/Controlled Current Source  Commented=on  Initialize=on  Source_Type=AC  Amplitude=0  Phase=0  Frequency=0  Measurements=None
  DP --> EMT : Subsystem  Commented=on
  Dynamic Phasor coeficients extraction : Subsystem  Commented=on
  Freq : Step  Time=2.8  After=-2  SampleTime=Ts
  Freq Ref : Step  Time=2  Before=60  After=58  SampleTime=Ts
  Ground1 : spsGroundLib/Ground  Commented=on  LConnTagsString=a
  Mux1 : Mux  Inputs=3
  Phase Ref : Constant  Value=0  SampleTime=Ts
  Phasor_to_Time_Domain_SFA : Subsystem  mask(Time domain from Dynamic Phasor){offset=60}
      mask prompts: offset "Frequency shift"
      mask help: This block extracts Time Domain Signals from the Dynamic Phasor by using the SFA method. It is usable only for three-phase signals
  Scope : Scope
  Series RLC Branch : spsSeriesRLCBranchLib/Series RLC Branch  Commented=on  LConnTagsString=__new0  RConnTagsString=__new0  BranchType=R  Resistance=0.5  Inductance=1e-3  SetiL0=off  InitialCurrent=0  Capacitance=1e-6  Setx0=off  InitialVoltage=0  Measurements=None
  Sum : Sum  Inputs=-+|
  Sum1 : Sum  Inputs=|+-
  Three-Phase Series RLC Branch1 : spsThreePhaseSeriesRLCBranchLib/Three-Phase Series RLC Branch  LConnTagsString=A|B|C  RConnTagsString=A|B|C  BranchType=R  Resistance=2  Inductance=1e-3  Capacitance=1e-6  Measurements=None
  Three-Phase V-I Measurement : spsThreePhaseVIMeasurementLib/Three-Phase V-I Measurement  VoltageMeasurement=phase-to-ground  SetLabelV=off  LabelV=Vabc  Vpu=off  VpuLL=off  CurrentMeasurement=yes  SetLabelI=off  LabelI=Iabc  Ipu=off  Pbase=100e6  Vbase=25e3  OutputType=Complex  PhasorSimulation=off  PSBequivalent=0
  Three-Phase Controlled Y-Connected Current Source : Subsystem
      settings: PortSchema="{\"entries\":[{\"content\":{\"sides\":[{\"content\":{\"connectorIds\":[\"LConn1\",\"LConn2\",\"LConn3\"]},\"type\":\"ConnectorPlacement.EquallySpacedRectSide\",\"uuid\":\"a8a67328-a09d-4495-b33c-aaf3ca0795cb\"},{\"content\":{\"connectorIds\":[\"In1\",\"In2\",\"In3\"],\"side\":\"RIGHT\"},\"type\":\"ConnectorPlacement.EquallySpacedRectSide\",\"uuid\":\"ca8d97e2-0dea-49aa-8cb7-235b4eace1f8\"},{\"content\":{\"connectorIds\":[],\"side\":\"TOP\"},\"type\":\"ConnectorPlacement.EquallySpacedRectSide\",\"uuid\":\"ab6aade9-1d27-4135-8ce1-c4358d4ecc87\"}]},\"type\":\"ConnectorPlacement.EquallySpacedConnector\",\"uuid\":\"205b5c38-55ea-4d68-a706-de660c21807c\"}],\"packageUris\":[\"http://schema.mathworks.com/mf0/Connector/19700101\"],\"version\":\"1.0\"}"
  Time_Domain_To_Phasor_SFA : Subsystem  mask(SFA){offset=60}
      mask prompts: offset "Frequency shift"
      mask help: This block extracts Dynamic Phasor by using the SFA method. It is usable only for three-phase signals
  Voltage Measurement : spsVoltageMeasurementLib/Voltage Measurement  Commented=on  PhasorSimulation=off  OutputType=Complex  PSBequivalent=0
  Vabc_Phasor_out : Outport
  I_injected : Outport  Port=2
  wires:
  DP --> EMT/1(I_injected) -> Controlled Current Source/1
  Voltage Measurement/1 -> Dynamic Phasor coeficients extraction/1(EMT Signal)
  Data_In/1 -> Phasor_to_Time_Domain_SFA/1(Dynamic_Phasor)
  Three-Phase V-I Measurement/1 -> Scope/1, Time_Domain_To_Phasor_SFA/1(EMT)
  Time_Domain_To_Phasor_SFA/1(Dynamic_Phasor) -> Vabc_Phasor_out/1
  Phasor_to_Time_Domain_SFA/1(A) -> Mux1/1, Three-Phase Controlled Y-Connected Current Source/1(Ia)
  Mux1/1 -> I_injected/1
  Phasor_to_Time_Domain_SFA/2(B) -> Mux1/2, Three-Phase Controlled Y-Connected Current Source/2(Ib)
  Phasor_to_Time_Domain_SFA/3(C) -> Mux1/3, Three-Phase Controlled Y-Connected Current Source/3(Ic)
  Phase Ref/1 -> "Controllable Voltage Source "/2(Phase [Deg])
  Amplitude/1 -> Sum/2
  Sum/1 -> "Controllable Voltage Source "/1(Amplitude [V])
  "Amplitude1 "/1 -> Sum/1
  Freq Ref/1 -> Sum1/1
  Sum1/1 -> "Controllable Voltage Source "/3(Frequency [Hz])
  Freq/1 -> Sum1/2
  connections:
  AC Voltage Source/RConn1 -- Series RLC Branch/LConn1
  AC Voltage Source/LConn1 -- Controlled Current Source/RConn1 -- Voltage Measurement/LConn2 -- Ground1/LConn1
  Series RLC Branch/RConn1 -- Voltage Measurement/LConn1 -- Controlled Current Source/LConn1
  Three-Phase Series RLC Branch1/RConn2 -- Three-Phase V-I Measurement/LConn2
  Three-Phase V-I Measurement/LConn3 -- Three-Phase Series RLC Branch1/RConn3
  Three-Phase V-I Measurement/LConn1 -- Three-Phase Series RLC Branch1/RConn1
  Three-Phase Controlled Y-Connected Current Source/LConn1 -- Three-Phase V-I Measurement/RConn1
  Three-Phase V-I Measurement/RConn2 -- Three-Phase Controlled Y-Connected Current Source/LConn2
  Three-Phase V-I Measurement/RConn3 -- Three-Phase Controlled Y-Connected Current Source/LConn3
  "Controllable Voltage Source "/RConn1 -- Three-Phase Series RLC Branch1/LConn1
  "Controllable Voltage Source "/RConn2 -- Three-Phase Series RLC Branch1/LConn2
  "Controllable Voltage Source "/RConn3 -- Three-Phase Series RLC Branch1/LConn3

== system basic_cosimulation_c_1_sm_master/SM_Master/OpComm ==
  Demux : Demux  Outputs="[1  2]"
  Receive : opal_lib/Communication/OpRecPar FromNT  Data_width=3  InitialConditions=[0;0;0]
  busStruct : Subsystem
  Out1 : Outport
  Out2 : Outport  Port=2
  wires:
  Demux/2 -> busStruct/2(In2)
  Demux/1 -> busStruct/1(In1)
  busStruct/2(Out2) -> Out2/1
  busStruct/1(Out1) -> Out1/1
  Receive/1 -> Demux/1

== system basic_cosimulation_c_1_sm_master/SM_Master/Original Circuit ==
  note: Inverter Measurements
  note: Model Control
  dblk : Inport
  PQ_ref : Inport  Port=2
  ARTEMiS SSN IVIC : ssn_inverter_model/ARTEMiS SSN IVIC  Arms=3  SnubberResistance=800  SnubberCapacitance=inf  Device=IGBT / Diodes  Ron=1e-3  Lon=0  ForwardVoltages=[0.001 0.001]  ForwardVoltage=0  GTOparameters=[ 10e-6 , 20e-6 ]  IGBTparameters=[ 1e-6 , 2e-6 ]*0  Measurements=None  Measurements_2=None  converterType=Rectifier
  Control : Subsystem
      settings: PortSchema="{\"entries\":[{\"content\":{\"sides\":[{\"content\":{\"connectorIds\":[\"In1\",\"In2\",\"In3\",\"In4\"]},\"type\":\"ConnectorPlacement.EquallySpacedRectSide\",\"uuid\":\"9324a1b5-9209-40a7-bba6-3b17f55cd5b4\"},{\"content\":{\"connectorIds\":[\"Out1\"],\"side\":\"RIGHT\"},\"type\":\"ConnectorPlacement.EquallySpacedRectSide\",\"uuid\":\"8b60fbd3-efee-4b93-84ca-13d5af533164\"},{\"content\":{\"connectorIds\":[],\"side\":\"TOP\"},\"type\":\"ConnectorPlacement.EquallySpacedRectSide\",\"uuid\":\"5aa46534-718a-472c-a25f-19e1867ae9eb\"},{\"content\":{\"connectorIds\":[\"Out2\"],\"side\":\"BOTTOM\"},\"type\":\"ConnectorPlacement.EquallySpacedRectSide\",\"uuid\":\"4a562f23-b1c9-4bd2-8d21-c9ff01dab3f7\"},{\"content\":{\"connectorIds\":[],\"side\":\"HIDDEN\"},\"type\":\"ConnectorPlacement.EquallySpacedRectSide\",\"uuid\":\"2bae700d-a0ed-419d-b89d-d5ddfcfc4dca\"}]},\"type\":\"ConnectorPlacement.EquallySpacedConnector\",\"uuid\":\"0ed67f90-7cb8-4c5b-bc99-423fd2f61638\"}],\"packageUris\":[\"http://schema.mathworks.com/mf0/Connector/R2020b\"],\"version\":\"1.0\"}"
  Current Measurement{,1..2,6} (4 alike) : spsCurrentMeasurementLib/Current Measurement  PhasorSimulation=off  OutputType=Complex  PSBequivalent=0
  DC Voltage Source : spsDCVoltageSourceLib/DC Voltage Source  Amplitude=Vdc  Measurements=None
  Delay : Delay  DelayLength=1
  Delay1 : Delay  DelayLength=1
  Delay2 : Delay  DelayLength=1
  Demux : Demux  Outputs=10
  Filter Capacitor : spsThreePhaseSeriesRLCBranchLib/Three-Phase Series RLC Branch  LConnTagsString=A|B|C  RConnTagsString=A|B|C  BranchType=RC  Resistance=Rf  Inductance=L_inv  Capacitance=Cf  Measurements=None
  Filter Inductor : spsThreePhaseSeriesRLCBranchLib/Three-Phase Series RLC Branch  LConnTagsString=A|B|C  RConnTagsString=A|B|C  BranchType=RL  Resistance=1e-3  Inductance=L_inv  Capacitance=1e-6  Measurements=None
  Iabc : Scope  NumInputPorts=3
  Icc_in : Scope
  Idq : Scope  NumInputPorts=2
  Mux : Mux  Inputs=2
  Mux1 : Mux  Inputs=3
  Mux2 : Mux  Inputs=6
  PWM : Subsystem  AncestorBlock=LafaeLib/PV System/PV System Detailed/VSC_Control/PWM
  Three-Phase Transformer (Two Windings) : spsThreePhaseTransformerTwoWindingsLib/Three-Phase Transformer (Two Windings)  Winding1Connection=Delta (D1)  Winding2Connection=Yg  CoreType=Three single-phase transformers  SetSaturation=off  Hysteresis=off  DataFile='hysteresis'  SetInitialFlux=off  Measurements=None  UNITS=pu  NominalPower=[ 80e3 , 60 ]  Winding1=[ Vnom_rms*sqrt(3) , 0.002 , 0.02 ]  Winding2=[440 , 0.002 , 0.02 ]  Rm=500  Lm=500  L0=0.5  Saturation=[ 0,0 ; 0.0024,1.2 ; 1.0,1.52 ]  InitialFluxes=[ 0.8 , -0.8 , 0.7 ]  BreakLoop=off  DiscreteSolver=Trapezoidal iterative  DataType=off  TransfoNumber=1
  Three-Phase Source : spsThreePhaseSourceLib/Three-Phase Source  InternalConnection=Yg  VoltagePhases=off  Voltage=440  PhaseAngle=0  Voltage_phases=[25e3 25e3 25e3]/sqrt(3)  PhaseAngles_phases=[0 -120 +120]  Frequency=60  NonIdealSource=on  SpecifyImpedance=off  Resistance=0.1e-3  Inductance=0.1e-3  ShortCircuitLevel=100e6  BaseVoltage=440  XRratio=7  BusType=swing  Pref=10e3  Qref=0  Prefabc=[10e3, 10e3, 10e3]  Qrefabc=[0, 0, 0]  Qmin=-inf  Qmax=inf
  Universal Bridge : spsUniversalBridgeLib/Universal Bridge  Commented=on  Arms=3  SnubberResistance=1e5  SnubberCapacitance=inf  Device=Average-model based VSC  Ron=1e-3  Lon=0  ForwardVoltages="[  0  0  ]"  ForwardVoltage=0  GTOparameters=[ 10e-6 , 20e-6 ]  IGBTparameters=[ 1e-6 , 2e-6 ]  Measurements=None  Measurements_2=None  converterType=Rectifier
  Vabc : Scope  NumInputPorts=3
  Vdq : Scope  NumInputPorts=2
  Voltage Measurement1 : spsVoltageMeasurementLib/Voltage Measurement  PhasorSimulation=off  OutputType=Complex  PSBequivalent=0
  Voltage Measurement2 : spsVoltageMeasurementLib/Voltage Measurement  PhasorSimulation=off  OutputType=Complex  PSBequivalent=0
  REF_V_I : Outport
  wires:
  dblk/1 -> [dblk]
  PQ_ref/1 -> [PQ_ref]
  Voltage Measurement1/1 -> Delay1/1
  Voltage Measurement2/1 -> Delay/1
  Current Measurement6/1 -> Icc_in/1
  Demux/1 -> Idq/1
  Control/1(Mabc) -> PWM/1(Uabc_ref)
  Delay1/1 -> [Vbc]
  Current Measurement/1 -> [ia]
  [dblk] -> Control/3(Deblock_inv)
  Demux/10 -> Mux2/6, Vabc/3
  Delay/1 -> [Vab]
  [Vab] -> Mux/1
  Delay2/1 -> Control/2(Iabc)
  [meas] -> Demux/1
  Demux/9 -> Mux2/5, Vabc/2
  Demux/2 -> Idq/2
  Demux/8 -> Vabc/1, Mux2/4
  Demux/3 -> Mux2/1, Iabc/1
  Demux/7 -> Vdq/2
  [ia] -> Mux1/1
  Control/2(Measures) -> [meas]
  [ib] -> Mux1/2
  [PQ_ref] -> Control/4(PQ_ref)
  Mux/1 -> Control/1(Vline)
  Demux/6 -> Vdq/1
  [Vbc] -> Mux/2
  Mux1/1 -> Delay2/1
  Demux/5 -> Iabc/3, Mux2/3
  Current Measurement2/1 -> [ic]
  Current Measurement1/1 -> [ib]
  [ic] -> Mux1/3
  PWM/1(Uref) -> ARTEMiS SSN IVIC/1
  Demux/4 -> Mux2/2, Iabc/2
  Mux2/1 -> REF_V_I/1
  connections:
  Filter Capacitor/LConn3 -- Voltage Measurement1/LConn2 -- Three-Phase Transformer (Two Windings)/LConn3 -- Current Measurement2/RConn1
  Filter Capacitor/RConn1 -- Filter Capacitor/RConn2 -- Filter Capacitor/RConn3
  Voltage Measurement1/LConn1 -- Three-Phase Transformer (Two Windings)/LConn2 -- Current Measurement1/RConn1 -- Filter Capacitor/LConn2 -- Voltage Measurement2/LConn2
  Three-Phase Transformer (Two Windings)/LConn1 -- Current Measurement/RConn1 -- Filter Capacitor/LConn1 -- Voltage Measurement2/LConn1
  Three-Phase Transformer (Two Windings)/RConn2 -- Three-Phase Source/RConn2
  DC Voltage Source/RConn1 -- Current Measurement6/LConn1
  Three-Phase Transformer (Two Windings)/RConn3 -- Three-Phase Source/RConn3
  Three-Phase Transformer (Two Windings)/RConn1 -- Three-Phase Source/RConn1
  ARTEMiS SSN IVIC/RConn2 -- DC Voltage Source/LConn1
  Current Measurement1/LConn1 -- Filter Inductor/RConn2
  Current Measurement6/RConn1 -- ARTEMiS SSN IVIC/RConn1
  ARTEMiS SSN IVIC/LConn2 -- Filter Inductor/LConn2
  ARTEMiS SSN IVIC/LConn1 -- Filter Inductor/LConn1
  Current Measurement2/LConn1 -- Filter Inductor/RConn3
  ARTEMiS SSN IVIC/LConn3 -- Filter Inductor/LConn3
  Current Measurement/LConn1 -- Filter Inductor/RConn1

== system basic_cosimulation_c_1_sm_master/SM_Master/Original_Circuit ==
  Amplitude : Step  Time=3  Before=220*sqrt(2/3)  After=220*sqrt(2/3)  SampleTime=Ts
  "Amplitude1 " : Step  Time=4  After=0  SampleTime=Ts
  "Controllable Voltage Source " : Subsystem
  Freq : Step  Time=2.8  After=0  SampleTime=Ts
  Freq Ref : Step  Time=2  Before=60  After=60  SampleTime=Ts
  Ground : spsGroundLib/Ground  LConnTagsString=a
  Mux : Mux  Inputs=2
  Phase Ref : Constant  Value=0  SampleTime=Ts
  Sum : Sum  Inputs=-+|
  Sum1 : Sum  Inputs=|+-
  Three-Phase Series RLC Branch : spsThreePhaseSeriesRLCBranchLib/Three-Phase Series RLC Branch  LConnTagsString=A|B|C  RConnTagsString=A|B|C  BranchType=RL  Resistance=5  Inductance=1e-3  Capacitance=1e-6  Measurements=None
  Three-Phase Series RLC Branch1 : spsThreePhaseSeriesRLCBranchLib/Three-Phase Series RLC Branch  LConnTagsString=A|B|C  RConnTagsString=A|B|C  BranchType=R  Resistance=2  Inductance=1e-3  Capacitance=1e-6  Measurements=None
  Three-Phase V-I Measurement1 : spsThreePhaseVIMeasurementLib/Three-Phase V-I Measurement  VoltageMeasurement=phase-to-ground  SetLabelV=off  LabelV=Vabc  Vpu=off  VpuLL=off  CurrentMeasurement=yes  SetLabelI=off  LabelI=Iabc  Ipu=off  Pbase=100e6  Vbase=25e3  OutputType=Complex  PhasorSimulation=off  PSBequivalent=0
  Three-Phase Breaker : spsThreePhaseBreakerLib/Three-Phase Breaker  InitialState=open  SwitchA=on  SwitchB=on  SwitchC=on  SwitchTimes=[1]  External=off  BreakerResistance=0.001  SnubberResistance=1e6  SnubberCapacitance=inf  Measurements=None
  Vabc_Iabc_original : Outport
  wires:
  Three-Phase V-I Measurement1/1 -> Mux/1
  Three-Phase V-I Measurement1/2 -> Mux/2
  Mux/1 -> Vabc_Iabc_original/1
  Freq Ref/1 -> Sum1/1
  Sum/1 -> "Controllable Voltage Source "/1(Amplitude [V])
  Phase Ref/1 -> "Controllable Voltage Source "/2(Phase [Deg])
  Freq/1 -> Sum1/2
  Sum1/1 -> "Controllable Voltage Source "/3(Frequency [Hz])
  Amplitude/1 -> Sum/2
  "Amplitude1 "/1 -> Sum/1
  connections:
  Three-Phase V-I Measurement1/LConn2 -- Three-Phase Series RLC Branch1/RConn2
  Three-Phase V-I Measurement1/LConn1 -- Three-Phase Series RLC Branch1/RConn1
  Three-Phase V-I Measurement1/LConn3 -- Three-Phase Series RLC Branch1/RConn3
  Ground/LConn1 -- Three-Phase Series RLC Branch/RConn1 -- Three-Phase Series RLC Branch/RConn3 -- Three-Phase Series RLC Branch/RConn2
  "Controllable Voltage Source "/RConn2 -- Three-Phase Series RLC Branch1/LConn2
  "Controllable Voltage Source "/RConn1 -- Three-Phase Series RLC Branch1/LConn1
  "Controllable Voltage Source "/RConn3 -- Three-Phase Series RLC Branch1/LConn3
  Three-Phase Breaker/LConn1 -- Three-Phase V-I Measurement1/RConn1
  Three-Phase Breaker/LConn2 -- Three-Phase V-I Measurement1/RConn2
  Three-Phase Breaker/LConn3 -- Three-Phase V-I Measurement1/RConn3
  Three-Phase Breaker/RConn1 -- Three-Phase Series RLC Branch/LConn1
  Three-Phase Breaker/RConn2 -- Three-Phase Series RLC Branch/LConn2
  Three-Phase Breaker/RConn3 -- Three-Phase Series RLC Branch/LConn3

== system basic_cosimulation_c_1_sm_master/SM_Master/Saving RT Data ==
  group26 : Inport
  group27 : Inport  Port=2
  group28 : Inport  Port=3
  group29 : Inport  Port=4
  Bus to Vector{1..4} (4 alike) : BusToVector
  OpWriteFile26 : rtlab/DataLogging/OpWriteFile  Static_File=on  varname=data_send  Filename=data_send.mat  rtpath='./'  nrtpath='.\'  Acq_Group=26  file_size=(nls26+1)*8*(ld26/Ts)*1.5  write_offline=on  Sim_Mode=off  Nb_Samples=ld26/Ts  Buffer_size=(ld26/Ts)*8*(1+nls26)
      settings: SourceProductName=RT-LAB
  OpWriteFile27 : rtlab/DataLogging/OpWriteFile  Static_File=on  varname=data_recv  Filename=data_recv.mat  rtpath='./'  nrtpath='.\'  Acq_Group=27  file_size=(nls27+1)*8*(ld27/Ts)*1.5  write_offline=on  Sim_Mode=off  Nb_Samples=ld27/Ts  Buffer_size=(ld26/Ts)*8*(1+nls26)
      settings: SourceProductName=RT-LAB
  OpWriteFile28 : rtlab/DataLogging/OpWriteFile  Static_File=on  varname=I_injected  Filename=I_injected.mat  rtpath='./'  nrtpath='.\'  Acq_Group=28  file_size=(nls28+1)*8*(ld28/Ts)*1.5  write_offline=on  Sim_Mode=off  Nb_Samples=ld28/Ts  Buffer_size=(ld28/Ts)*8*(1+nls28)
      settings: SourceProductName=RT-LAB
  OpWriteFile29 : rtlab/DataLogging/OpWriteFile  Static_File=on  varname=Ref_V_I  Filename=Ref_V_I.mat  rtpath='./'  nrtpath='.\'  Acq_Group=29  file_size=(nls29+1)*8*(ld29/Ts)*1.5  write_offline=on  Sim_Mode=off  Nb_Samples=ld29/Ts  Buffer_size=(ld29/Ts)*8*(1+nls29)
      settings: SourceProductName=RT-LAB
  Terminator{1..8} (8 alike) : Terminator
  wires:
  OpWriteFile28/2 -> Terminator6/1
  OpWriteFile27/1 -> Terminator1/1
  OpWriteFile26/2 -> Terminator3/1
  OpWriteFile26/1 -> Terminator2/1
  OpWriteFile27/2 -> Terminator4/1
  OpWriteFile29/2 -> Terminator8/1
  OpWriteFile29/1 -> Terminator7/1
  OpWriteFile28/1 -> Terminator5/1
  group26/1 -> [group26]
  group27/1 -> [group27]
  group28/1 -> [group28]
  group29/1 -> [group29]
  [group27] -> Bus to Vector1/1
  Bus to Vector1/1 -> OpWriteFile27/1
  [group29] -> Bus to Vector2/1
  Bus to Vector2/1 -> OpWriteFile29/1
  [group26] -> Bus to Vector3/1
  Bus to Vector3/1 -> OpWriteFile26/1
  [group28] -> Bus to Vector4/1
  Bus to Vector4/1 -> OpWriteFile28/1
